simulink model "mdl4"  (Simulink 8.3)
settings: Solver=FixedStepDiscrete  SolverMode=SingleTasking  StartTime=TIME(1)  StopTime=TIME(end)  FixedStep=SIMSTEP  RelTol=1e-3
values from neighbouring files (symbols this model uses):
  Parameter113 = 123    [scr_simdata_all.mat]
  Parameter131 = 3    [scr_simdata_all.mat]
  Parameter132 = 100    [scr_simdata_all.mat]
  Parameter144 = 3    [scr_simdata_all.mat]
  Parameter51 = 0    [scr_simdata_all.mat]
  Parameter52 = 1    [scr_simdata_all.mat]
  Parameter53 = 2    [scr_simdata_all.mat]
  Parameter54 = 255    [scr_simdata_all.mat]
  Parameter69 = 27    [scr_simdata_all.mat]
  Parameter91 = 75    [scr_simdata_all.mat]
  SIMSTEP = 0.0001024    [scr_simdata_all.mat]
(part 4 of 4)

== system mdl4/SubSystem2493/SubSystem2494/SubSystem2500/SubSystem2504/SubSystem2533/SubSystem2567/SubSystem2574 ==
  note: Text665
  note: Text664
  note: Text663
  note: Text662
  note: Text661
  Block7694 : Inport
  Block7695 : TriggerPort  TriggerType=function-call
  Block7696 : DataStoreRead  DataStoreName=DSM288
  Block7697 : DataStoreRead  DataStoreName=DSM287
  Block7698 : DataStoreWrite  DataStoreName=DSM288
  Block7699 : DataStoreWrite  DataStoreName=DSM287
  Block7700 : Sum  Inputs=++|  OutDataTypeStr=double  RndMeth=Zero  SaturateOnIntegerOverflow=on  InputSameDT=on
  Block7701 : Sum  Inputs=++|  OutDataTypeStr=double  RndMeth=Zero  SaturateOnIntegerOverflow=on  InputSameDT=on
  SubSystem2575 : Subsystem  TreatAsAtomicUnit=on  mask(***ATC.DSRVEC***){bd_version=1.01.A, r0=DSM281, r1=-1, r2=, r3=, r4=, r5=, r6=, r7=, r8=, r9=, c0=, c1=, c2=, c3=, c4=, c5=, c6=, c7=, c8=, c9=}
      mask prompts: bd_version "Version"
      mask help: これはAutoCからのブロックです．編集禁止．
      settings: OpenFcn=warndlg('変更禁止!');
      mask Help: web(ui_blockhelpmng(gcb));
      mask Display: disp('ATC.DSRVEC')
  SubSystem2576 : Subsystem  TreatAsAtomicUnit=on  mask(***ATC.DSRVEC***){bd_version=1.01.A, r0=DSM282, r1=-1, r2=, r3=, r4=, r5=, r6=, r7=, r8=, r9=, c0=, c1=, c2=, c3=, c4=, c5=, c6=, c7=, c8=, c9=}
      mask prompts: bd_version "Version"
      mask help: これはAutoCからのブロックです．編集禁止．
      settings: OpenFcn=warndlg('変更禁止!');
      mask Help: web(ui_blockhelpmng(gcb));
      mask Display: disp('ATC.DSRVEC')
  wires:
  Block7700/1 -> Block7698/1  "mdl4_SubSystem2493_SubSystem2494_SubSystem2500_SubSystem2504_SubSystem2533_SubSystem2567_SubSystem2574_Block7700_1"
  Block7696/1 -> Block7700/1  "mdl4_SubSystem2493_SubSystem2494_SubSystem2500_SubSystem2504_SubSystem2533_SubSystem2567_SubSystem2574_Block7696_1"
  Block7701/1 -> Block7699/1  "mdl4_SubSystem2493_SubSystem2494_SubSystem2500_SubSystem2504_SubSystem2533_SubSystem2567_SubSystem2574_Block7701_1"
  Block7697/1 -> Block7701/1  "mdl4_SubSystem2493_SubSystem2494_SubSystem2500_SubSystem2504_SubSystem2533_SubSystem2567_SubSystem2574_Block7697_1"
  SubSystem2575/1(Output) -> Block7701/2  "mdl4_SubSystem2493_SubSystem2494_SubSystem2500_SubSystem2504_SubSystem2533_SubSystem2567_SubSystem2574_SubSystem2575_SigLabel299"
  Block7694/1 -> SubSystem2575/1(element), SubSystem2576/1(element)
  SubSystem2576/1(Output) -> Block7700/2  "mdl4_SubSystem2493_SubSystem2494_SubSystem2500_SubSystem2504_SubSystem2533_SubSystem2567_SubSystem2574_SubSystem2576_SigLabel298"

== system mdl4/SubSystem2493/SubSystem2494/SubSystem2500/SubSystem2504/SubSystem2533/SubSystem2547/SubSystem2554/SubSystem2555 ==
  note: ***編集禁止***
  element : Inport
  Inside_DSR : DataStoreRead  DataStoreName=DSM293
  Selector : Selector  IndexOptions=Index vector (port)  Indices=[1 3]
  Output : Outport
  wires:
  Inside_DSR/1 -> Selector/1  "mdl4_SubSystem2493_SubSystem2494_SubSystem2500_SubSystem2504_SubSystem2533_SubSystem2547_SubSystem2554_SubSystem2555_Inside_DSR_1"
  element/1 -> Selector/2
  Selector/1 -> Output/1

== system mdl4/SubSystem2493/SubSystem2494/SubSystem2500/SubSystem2504/SubSystem2533/SubSystem2547/SubSystem2554/SubSystem2556 ==
  note: ***編集禁止***
  element : Inport
  Inside_DSR : DataStoreRead  DataStoreName=DSM295
  Selector : Selector  IndexOptions=Index vector (port)  Indices=[1 3]
  Output : Outport
  wires:
  Selector/1 -> Output/1
  element/1 -> Selector/2
  Inside_DSR/1 -> Selector/1  "mdl4_SubSystem2493_SubSystem2494_SubSystem2500_SubSystem2504_SubSystem2533_SubSystem2547_SubSystem2554_SubSystem2556_Inside_DSR_1"

== system mdl4/SubSystem2493/SubSystem2494/SubSystem2500/SubSystem2504/SubSystem2533/SubSystem2557/SubSystem2564/SubSystem2565 ==
  note: ***編集禁止***
  element : Inport
  Inside_DSR : DataStoreRead  DataStoreName=DSM279
  Selector : Selector  IndexOptions=Index vector (port)  Indices=[1 3]
  Output : Outport
  wires:
  Inside_DSR/1 -> Selector/1  "mdl4_SubSystem2493_SubSystem2494_SubSystem2500_SubSystem2504_SubSystem2533_SubSystem2557_SubSystem2564_SubSystem2565_Inside_DSR_1"
  element/1 -> Selector/2
  Selector/1 -> Output/1

== system mdl4/SubSystem2493/SubSystem2494/SubSystem2500/SubSystem2504/SubSystem2533/SubSystem2557/SubSystem2564/SubSystem2566 ==
  note: ***編集禁止***
  element : Inport
  Inside_DSR : DataStoreRead  DataStoreName=DSM280
  Selector : Selector  IndexOptions=Index vector (port)  Indices=[1 3]
  Output : Outport
  wires:
  Selector/1 -> Output/1
  element/1 -> Selector/2
  Inside_DSR/1 -> Selector/1  "mdl4_SubSystem2493_SubSystem2494_SubSystem2500_SubSystem2504_SubSystem2533_SubSystem2557_SubSystem2564_SubSystem2566_Inside_DSR_1"

== system mdl4/SubSystem2493/SubSystem2494/SubSystem2500/SubSystem2504/SubSystem2533/SubSystem2567/SubSystem2574/SubSystem2575 ==
  note: ***編集禁止***
  element : Inport
  Inside_DSR : DataStoreRead  DataStoreName=DSM281
  Selector : Selector  IndexOptions=Index vector (port)  Indices=[1 3]
  Output : Outport
  wires:
  Inside_DSR/1 -> Selector/1  "mdl4_SubSystem2493_SubSystem2494_SubSystem2500_SubSystem2504_SubSystem2533_SubSystem2567_SubSystem2574_SubSystem2575_Inside_DSR_1"
  element/1 -> Selector/2
  Selector/1 -> Output/1

== system mdl4/SubSystem2493/SubSystem2494/SubSystem2500/SubSystem2504/SubSystem2533/SubSystem2567/SubSystem2574/SubSystem2576 ==
  note: ***編集禁止***
  element : Inport
  Inside_DSR : DataStoreRead  DataStoreName=DSM282
  Selector : Selector  IndexOptions=Index vector (port)  Indices=[1 3]
  Output : Outport
  wires:
  Selector/1 -> Output/1
  element/1 -> Selector/2
  Inside_DSR/1 -> Selector/1  "mdl4_SubSystem2493_SubSystem2494_SubSystem2500_SubSystem2504_SubSystem2533_SubSystem2567_SubSystem2574_SubSystem2576_Inside_DSR_1"

== stateflow chart SubSystem2493/SubSystem2494/SubSystem2500/SubSystem2504/SubSystem2533/SubSystem2557/SubSystem2563/For_loop ==
  note: for(i1 = 0; i1 < N_Loop; i1++) {
      |   処理
      | }
  (default) -> (junction 8) : {
      |  idx = 1;
      |  i1 = 0;
      | }
  (junction 9) -> (junction 8) : {i1++;}
  (junction 8) -> (junction 10)
  (junction 11) -> (junction 9) : {
      |  function_call;
      |  idx = idx + 1;
      | }
  (junction 10) -> (junction 11) [order 1] : [i1 < N_Loop]
  (junction 10) -> (junction 12) [order 2]
  data: N_Loop input double; i1 local int32; idx output int32
  events: function_call output FUNCTION_CALL_EVENT

== stateflow chart SubSystem2493/SubSystem2494/SubSystem2500/SubSystem2504/SubSystem2533/SubSystem2547/SubSystem2553/For_loop ==
  note: for(i1 = 0; i1 < N_Loop; i1++) {
      |   処理
      | }
  (default) -> (junction 26) : {
      |  idx = 1;
      |  i1 = 0;
      | }
  (junction 27) -> (junction 26) : {i1++;}
  (junction 26) -> (junction 28)
  (junction 29) -> (junction 27) : {
      |  function_call;
      |  idx = idx + 1;
      | }
  (junction 28) -> (junction 29) [order 1] : [i1 < N_Loop]
  (junction 28) -> (junction 30) [order 2]
  data: N_Loop input double; i1 local int32; idx output int32
  events: function_call output FUNCTION_CALL_EVENT

== stateflow chart SubSystem2493/SubSystem2494/SubSystem2500/SubSystem2504/SubSystem2533/SubSystem2567/SubSystem2573/For_loop ==
  note: for(i1 = 0; i1 < N_Loop; i1++) {
      |   処理
      | }
  (default) -> (junction 44) : {
      |  idx = 1;
      |  i1 = 0;
      | }
  (junction 45) -> (junction 44) : {i1++;}
  (junction 44) -> (junction 46)
  (junction 47) -> (junction 45) : {
      |  function_call;
      |  idx = idx + 1;
      | }
  (junction 46) -> (junction 47) [order 1] : [i1 < N_Loop]
  (junction 46) -> (junction 48) [order 2]
  data: N_Loop input double; i1 local int32; idx output int32
  events: function_call output FUNCTION_CALL_EVENT

== stateflow chart SubSystem2493/SubSystem2577/SubSystem2579/SubSystem2580/For_loop ==
  note: for(i1 = 0; i1 < N_Loop; i1++) {
      |   処理
      | }
  (default) -> (junction 62) : {
      |  idx = 1;
      |  i1 = 0;
      | }
  (junction 63) -> (junction 62) : {i1++;}
  (junction 62) -> (junction 64)
  (junction 65) -> (junction 63) : {
      |  function_call;
      |  idx = idx + 1;
      | }
  (junction 64) -> (junction 65) [order 1] : [i1 < N_Loop]
  (junction 64) -> (junction 66) [order 2]
  data: N_Loop input double; i1 local int32; idx output int32
  events: function_call output FUNCTION_CALL_EVENT
